simulink model "Duct_PressureLosstest"  (R2025a)
settings: Solver=VariableStepAuto  StartTime=0.0  StopTime=10.0  RelTol=1e-3
settings Model: Creator=ramch  LastModifiedBy=ramch

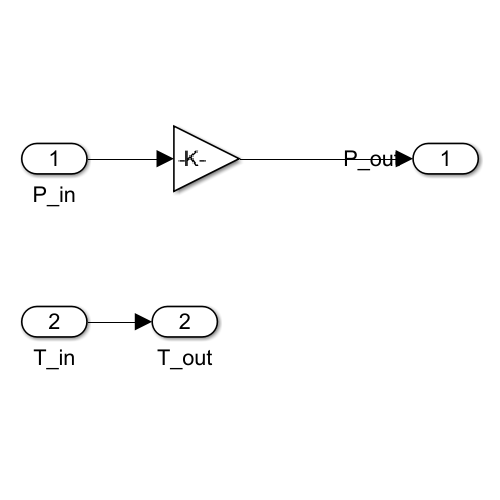
[thumbnail: Simulink's stored preview of the top-level diagram]
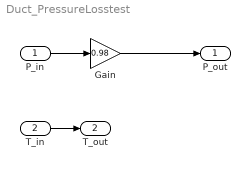
== system Duct_PressureLosstest ==
  P_in : Inport
  T_in : Inport  Port=2
  Gain : Gain  Gain=0.98
  P_out : Outport
  T_out : Outport  Port=2
  wires:
  P_in/1 -> Gain/1
  Gain/1 -> P_out/1
  T_in/1 -> T_out/1
